simulink library "trustRegion_ul"  (R2018a)
settings: Solver=VariableStepAuto  StartTime=0.0  StopTime=10.0  RelTol=1e-3
undefined symbols (not defined in the file or in its folder): ctrl
settings Model: Creator=mitch  LastModifiedBy=mitch

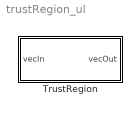
== system trustRegion_ul ==
  TrustRegion : Subsystem

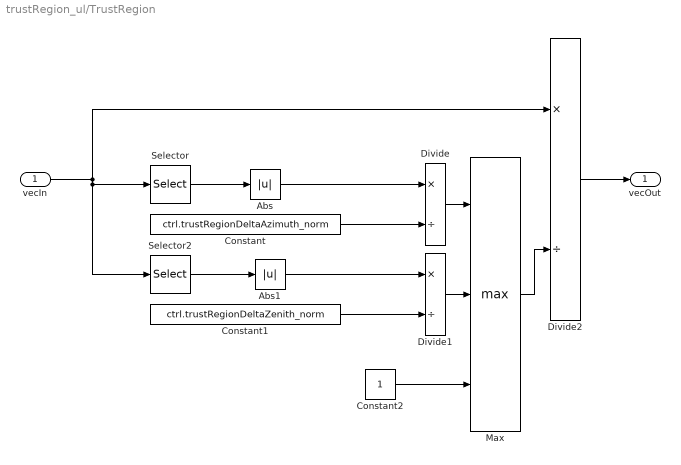
== system trustRegion_ul/TrustRegion ==
  vecIn : Inport
  Abs : Abs
  Abs1 : Abs
  Constant : Constant  Value=ctrl.trustRegionDeltaAzimuth_norm
  Constant1 : Constant  Value=ctrl.trustRegionDeltaZenith_norm
  Constant2 : Constant
  Divide : Product  Inputs=*/
  Divide1 : Product  Inputs=*/
  Divide2 : Product  Inputs=*/
  Max : MinMax  Function=max  Inputs=3
  Selector : Selector  InputPortWidth=2  IndexOptions=Index vector (dialog)  Indices=1  OutputSizes=1
  Selector2 : Selector  InputPortWidth=2  IndexOptions=Index vector (dialog)  Indices=2  OutputSizes=1
  vecOut : Outport
  wires:
  Selector/1 -> Abs/1
  Selector2/1 -> Abs1/1
  vecIn/1 -> Selector2/1, Selector/1, Divide2/1
  Divide/1 -> Max/1
  Divide1/1 -> Max/2
  Max/1 -> Divide2/2
  Divide2/1 -> vecOut/1
  Constant/1 -> Divide/2
  Constant1/1 -> Divide1/2
  Constant2/1 -> Max/3
  Abs/1 -> Divide/1
  Abs1/1 -> Divide1/1
